simulink library "SysGenQuantumLib"  (R2020b)
settings: Solver=VariableStepAuto  StartTime=0.0  StopTime=10.0  RelTol=1e-3
undefined symbols (not defined in the file or in its folder): AXI4, Lite
libraries: xbsIndex_r4 x4
settings Model: Creator=CDS-vmlynar  LastModifiedBy=CDS-vmlynar

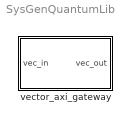
== system SysGenQuantumLib ==
  vector_axi_gateway : Subsystem  mask{WordWidth=16, FractionWidth=8, VecLen=4, BaseTs=8e-9, StartOffset=0, IntfName='cfg_in'}
      mask prompts: WordWidth "Number of bits"; FractionWidth "Number of fraction bits"; VecLen "Vector length"; BaseTs "Base sample time"; StartOffset "AXI interface starting offset"; IntfName "AXI interface name"
      mask init:
      | try
      |     set_param(gcb, 'LinkStatus', 'break');
      |     %disp(gcb)
      |     blocks = find_system(gcb,...
      |                 'LookUnderMasks','on',...
      |                 'FollowLinks','on',...
      |                 'MaskType','Xilinx Gateway In Block');
      | 
      |     if ~isempty(blocks)
      |         %disp(blocks)
      |         delete_block(blocks);
      |     end
      |     h_lines = find_system(gcb, 'FindAll', 'on','LookUnderMasks','on','FollowLinks','on', 'Type', 'line','Connected','off');
      | 
      |     if ~isempty(h_lines)
      |         delete_line(h_lines);
      |     end
      |     demux_block = find_system(gcb,...
      |                 'LookUnderMasks','on',...
      |                 'FollowLinks','on',...
      |                 'BlockType','Demux');
      |     %h_d_l = get_param(demux_block{1},'LineHandles');
      |     %if(~isempty(h_d_l))
      |     %    delete_line(h_d_l.Outport(:));
      |     %end
      |     set_param(demux_block{1},'Outputs','VecLen');
      |     h_d = get_param(demux_block{1},'PortHandles');
      |     
      |     mux_block = find_system(gcb,...
      |                 'LookUnderMasks','on',...
      |                 'FollowLinks','on',...
      |                 'BlockType','Mux');
      |     %h_m_l = get_param(mux_block{1},'LineHandles');
      |     %if(~isempty(h_m_l))
      |     %    delete_line(h_m_l.Inport(:));
      |     %end
      | 
      |     set_param(mux_block{1},'Inputs','VecLen');
      |     h_m = get_param(mux_block{1},'PortHandles');
      |     
      |     vec_in_inport = get_param([gcb,'/vec_in'],'PortConnectivity');
      |     
      |     % Prepare coordinates for block placement
      |     spacing = 25;
      |     XY_mid = vec_in_inport.Position; %Get center
      |     XY_top = XY_mid + [0 1]*round((VecLen*(spacing))/2);
      |     XY_bot = XY_mid - [0 1]*round((VecLen*(spacing))/2);
      |     
      |     for i = 1:VecLen
      |         h = add_block('XilinxModelComposer/HDL/Interfaces/Gateway In',[gcb,'/Gateway In'],'MakeNameUnique','on');
      |         set_param(h,'position',[-85, XY_bot(2)+i*spacing, -20, XY_bot(2)+20+i*spacing]);
      |         set_param(h,'n_bits', num2str(WordWidth),...
      |                     'bin_pt', num2str(FractionWidth),...
      |                     'arith_type', "Signed  (2's comp)",...
      |                     'gui_display_data_type', 'Fixed-point',...
      |                     'period', num2str(BaseTs),...
      |                     'Interface', 'AXI4-Lite',...
      |                     'automatic_assignment','off',...
      |                     'address_offset', "hex2dec('"+num2str(StartOffset+(i-1)*4,"%X")+"')",...
      |                     'intf_name', "'"+IntfName+"'");
      |         h_g = get_param(h,'PortHandles');
      | 
      |         add_line(gcb,h_d.Outport(i),h_g.Inport(1));
      |         add_line(gcb,h_g.Outport(1),h_m.Inport(i));
      |     end
      |     
      |     % Get the mask object
      |     mo = get_param(gcb,'MaskObject');
      |     % Get the text object
      |     tc = mo.getDialogControl('TextFinalAddress');
      |     % Change the string
      |     tc.Prompt = "Last relative address offset: 0x"+num2str((i-1)*4,"%X")+...
      |                 " from base address 0x"+num2str(StartOffset,"%X");
      |     
      |     %Simulink.BlockDiagram.arrangeSystem(gcb) 
      | catch ME
      |     disp(['Error while updating -> ' gcb])
      |     disp(ME.message)
      | end
      | %add_block('XilinxModelComposer/HDL/Interfaces/Gateway In',[gcb,'/Gateway In'],'MakeNameUnique','on');
      mask DialogControl ParameterGroupVar Prompt: Data type
      mask DialogControl Container3 Prompt: System parameters
      mask DialogControl TextFinalAddress Prompt: Last relative address offset: 0xC from base address 0x0

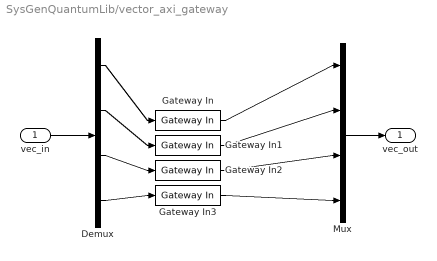
== system SysGenQuantumLib/vector_axi_gateway ==
  vec_in : Inport
  Demux : Demux  Outputs=VecLen
  Gateway In : xbsIndex_r4/Gateway In  gui_display_data_type=Fixed-point  arith_type="Signed  (2's comp)"  n_bits=16  bin_pt=8  preci_type=Single  exp_width=8  frac_width=24  rows=1  columns=1  quantization="Round  (unbiased: +/- Inf)"  overflow=Saturate  period=8e-09  UseAsADC=off  ADCChannel='1'  interface=AXI4-Lite  automatic_assignment=off  address_offset=hex2dec('0')  intf_name='cfg_in'  intf_description=''  default_value=0  timing_constraint=None  locs_specified=off  LOCs={}  io_standard={}  inherit_from_input=off  hdl_port=on  dbl_ovrd=off  block_type=gatewayin
  Gateway In1 : xbsIndex_r4/Gateway In  gui_display_data_type=Fixed-point  arith_type="Signed  (2's comp)"  n_bits=16  bin_pt=8  preci_type=Single  exp_width=8  frac_width=24  rows=1  columns=1  quantization="Round  (unbiased: +/- Inf)"  overflow=Saturate  period=8e-09  UseAsADC=off  ADCChannel='1'  interface=AXI4-Lite  automatic_assignment=off  address_offset=hex2dec('4')  intf_name='cfg_in'  intf_description=''  default_value=0  timing_constraint=None  locs_specified=off  LOCs={}  io_standard={}  inherit_from_input=off  hdl_port=on  dbl_ovrd=off  block_type=gatewayin
  Gateway In2 : xbsIndex_r4/Gateway In  gui_display_data_type=Fixed-point  arith_type="Signed  (2's comp)"  n_bits=16  bin_pt=8  preci_type=Single  exp_width=8  frac_width=24  rows=1  columns=1  quantization="Round  (unbiased: +/- Inf)"  overflow=Saturate  period=8e-09  UseAsADC=off  ADCChannel='1'  interface=AXI4-Lite  automatic_assignment=off  address_offset=hex2dec('8')  intf_name='cfg_in'  intf_description=''  default_value=0  timing_constraint=None  locs_specified=off  LOCs={}  io_standard={}  inherit_from_input=off  hdl_port=on  dbl_ovrd=off  block_type=gatewayin
  Gateway In3 : xbsIndex_r4/Gateway In  gui_display_data_type=Fixed-point  arith_type="Signed  (2's comp)"  n_bits=16  bin_pt=8  preci_type=Single  exp_width=8  frac_width=24  rows=1  columns=1  quantization="Round  (unbiased: +/- Inf)"  overflow=Saturate  period=8e-09  UseAsADC=off  ADCChannel='1'  interface=AXI4-Lite  automatic_assignment=off  address_offset=hex2dec('C')  intf_name='cfg_in'  intf_description=''  default_value=0  timing_constraint=None  locs_specified=off  LOCs={}  io_standard={}  inherit_from_input=off  hdl_port=on  dbl_ovrd=off  block_type=gatewayin
  Mux : Mux  Inputs=VecLen
  vec_out : Outport
  wires:
  vec_in/1 -> Demux/1
  Mux/1 -> vec_out/1
  Demux/1 -> Gateway In/1
  Gateway In/1 -> Mux/1
  Demux/2 -> Gateway In1/1
  Gateway In1/1 -> Mux/2
  Demux/3 -> Gateway In2/1
  Gateway In2/1 -> Mux/3
  Demux/4 -> Gateway In3/1
  Gateway In3/1 -> Mux/4
